simulink model "Rider_Controls_Control"  (R2014b)
settings: configuration reference "Embedded_Configuration" (kept outside this file)
PostLoadFcn:
  | load('Embedded_Config.mat')
model workspace: external: MAT-File C:\Users\Sean\Desktop\Buckeye Current\MagicSimNode\Rider_Controls.mat (data not in the file)
undefined symbols (not defined in the file or in its folder): alpha, BattTemp_Current_x, BattTemp_Current_y, RPM_Max_Current_x, RPM_Max_Current_y, SetPoint
libraries: simulink x1
settings Model: Creator=The MathWorks Inc.  LastModifiedBy=Sean

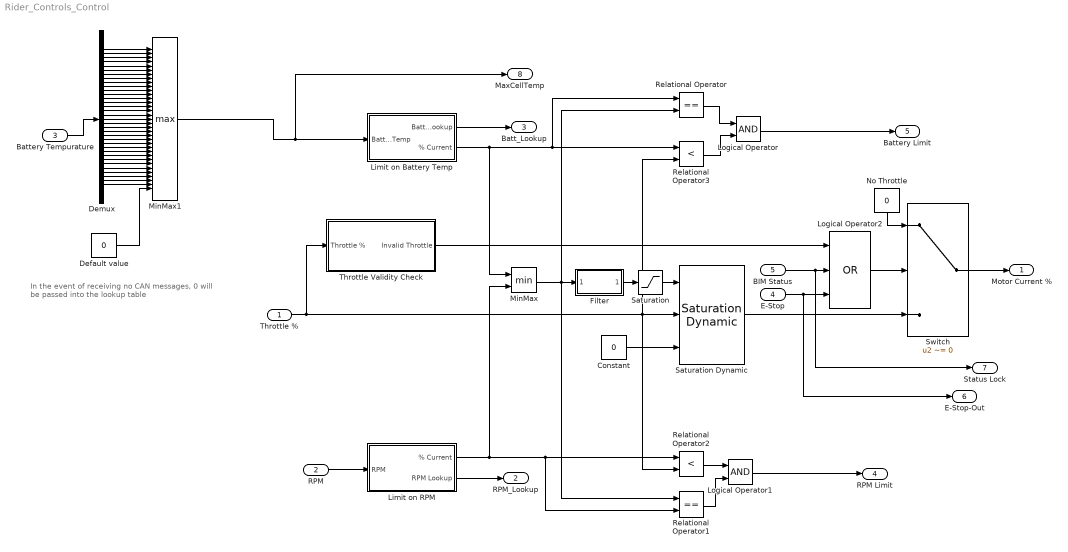
== system Rider_Controls_Control ==
  note: In the event of receiving no CAN messages,
      | 0 will be passed into the lookup table
  Throttle % : Inport  OutDataTypeStr=single  SampleTime=.01
  RPM : Inport  Port=2  OutDataTypeStr=single  SampleTime=.01
  Battery Tempurature : Inport  Port=3  OutDataTypeStr=single  SampleTime=.01
  E-Stop : Inport  Port=4
  BIM Status : Inport  Port=5
  Constant : Constant  Value=0  OutDataTypeStr=single
  Default value : Constant  Value=0  OutDataTypeStr=single
  Demux : Demux  Outputs=34
  Filter : Subsystem
  Limit on Battery Temp : Subsystem
  Limit on RPM : Subsystem
  Logical Operator : Logic  AllPortsSameDT=off  OutDataTypeStr=fixdt(0,16)
  Logical Operator1 : Logic  AllPortsSameDT=off  OutDataTypeStr=fixdt(0,16)
  Logical Operator2 : Logic  Operator=OR  Inputs=3  AllPortsSameDT=off  OutDataTypeStr=fixdt(0,16)
  MinMax : MinMax  Inputs=2
  MinMax1 : MinMax  Function=max  Inputs=35
  No Throttle : Constant  Value=0  OutDataTypeStr=single
  Relational Operator : RelationalOperator  Operator===  OutDataTypeStr=fixdt(0,16)
  Relational Operator1 : RelationalOperator  Operator===  OutDataTypeStr=fixdt(0,16)
  Relational Operator2 : RelationalOperator  Operator=<  OutDataTypeStr=fixdt(0,16)
  Relational Operator3 : RelationalOperator  Operator=<  OutDataTypeStr=fixdt(0,16)
  Saturation : Saturate  UpperLimit=1  LowerLimit=0
  Saturation Dynamic : simulink/Discontinuities/Saturation Dynamic  OutMin=[]  OutMax=[]  OutDataTypeStr=single  OutputDataTypeScalingMode=single  OutDataType=fixdt(1, 16)  OutScaling=2^-10  RndMeth=Nearest  DoSatur=off
  Switch : Switch  Criteria=u2 ~= 0
  Throttle Validity Check : Subsystem
  Motor Current % : Outport
  RPM_Lookup : Outport  Port=2  OutDataTypeStr=single  SampleTime=.01
  Batt_Lookup : Outport  Port=3  OutDataTypeStr=single
  "RPM Limit " : Outport  Port=4
  Battery Limit : Outport  Port=5
  "E-Stop-Out " : Outport  Port=6
  Status Lock : Outport  Port=7
  MaxCellTemp : Outport  Port=8
  wires:
  Throttle %/1 -> Throttle Validity Check/1(Throttle %), Relational Operator2/2, Relational Operator3/2, Saturation Dynamic/2
  Constant/1 -> Saturation Dynamic/3
  Saturation/1 -> Saturation Dynamic/1
  RPM/1 -> Limit on RPM/1(RPM)
  Limit on RPM/2(RPM Lookup) -> RPM_Lookup/1
  Limit on RPM/1(% Current) -> MinMax/2, Relational Operator2/1, Relational Operator1/2
  Limit on Battery Temp/2(% Current) -> MinMax/1, Relational Operator3/1, Relational Operator/1
  MinMax/1 -> Filter/1(Filter In), Relational Operator1/1, Relational Operator/2
  Limit on Battery Temp/1(Batt Temp Lookup) -> Batt_Lookup/1
  Relational Operator3/1 -> Logical Operator/2
  Relational Operator/1 -> Logical Operator/1
  Relational Operator2/1 -> Logical Operator1/1
  Relational Operator1/1 -> Logical Operator1/2
  No Throttle/1 -> Switch/1
  Saturation Dynamic/1 -> Switch/3
  Throttle Validity Check/1(Invalid Throttle) -> Logical Operator2/1
  Switch/1 -> Motor Current %/1
  BIM Status/1 -> Logical Operator2/2, Status Lock/1
  Battery Tempurature/1 -> Demux/1
  Demux/1 -> MinMax1/1
  Demux/2 -> MinMax1/2
  Demux/3 -> MinMax1/3
  Demux/4 -> MinMax1/4
  Demux/5 -> MinMax1/5
  Demux/6 -> MinMax1/6
  Demux/7 -> MinMax1/7
  Demux/8 -> MinMax1/8
  Demux/9 -> MinMax1/9
  Demux/10 -> MinMax1/10
  Demux/11 -> MinMax1/11
  Demux/12 -> MinMax1/12
  Demux/13 -> MinMax1/13
  Demux/14 -> MinMax1/14
  Demux/15 -> MinMax1/15
  Demux/16 -> MinMax1/16
  Demux/17 -> MinMax1/17
  Demux/18 -> MinMax1/18
  Demux/19 -> MinMax1/19
  Demux/20 -> MinMax1/20
  Demux/21 -> MinMax1/21
  Demux/22 -> MinMax1/22
  Demux/23 -> MinMax1/23
  Demux/24 -> MinMax1/24
  Demux/25 -> MinMax1/25
  Demux/26 -> MinMax1/26
  Demux/27 -> MinMax1/27
  Demux/28 -> MinMax1/28
  Demux/29 -> MinMax1/29
  Demux/30 -> MinMax1/30
  Demux/31 -> MinMax1/31
  Demux/32 -> MinMax1/32
  Demux/33 -> MinMax1/33
  Demux/34 -> MinMax1/34
  MinMax1/1 -> MaxCellTemp/1, Limit on Battery Temp/1(Battery Temp)
  E-Stop/1 -> "E-Stop-Out "/1, Logical Operator2/3
  Logical Operator2/1 -> Switch/2
  Logical Operator/1 -> Battery Limit/1
  Logical Operator1/1 -> "RPM Limit "/1
  Default value/1 -> MinMax1/35
  Filter/1(Filter Out) -> Saturation/1

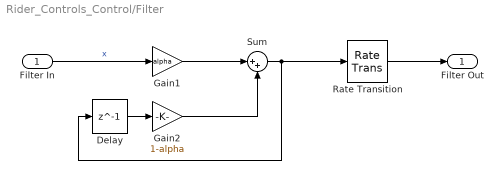
== system Rider_Controls_Control/Filter ==
  Filter In : Inport
  Delay : Delay  DelayLength=1
  Gain1 : Gain  Gain=alpha
  Gain2 : Gain  Gain=1-alpha
  Rate Transition : RateTransition  OutPortSampleTime=.01
  Sum : Sum  Inputs=|++  OutDataTypeStr=single
  Filter Out : Outport  SampleTime=.01
  wires:
  Rate Transition/1 -> Filter Out/1
  Sum/1 -> Delay/1, Rate Transition/1
  Gain2/1 -> Sum/2
  Delay/1 -> Gain2/1
  Gain1/1 -> Sum/1
  Filter In/1 -> Gain1/1  "x"

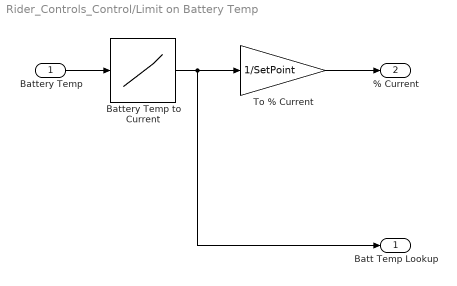
== system Rider_Controls_Control/Limit on Battery Temp ==
  Battery Temp : Inport
  Battery Temp to Current : Lookup_n-D  NumberOfTableDimensions=1  BreakpointsForDimension1=BattTemp_Current_x  BreakpointsForDimension1DataTypeStr=single  IndexSearchMethod=Linear search  BeginIndexSearchUsingPreviousIndexResult=on  Table=BattTemp_Current_y  TableDataTypeStr=single  IntermediateResultsDataTypeStr=single  RemoveProtectionInput=on  InternalRulePriority=Speed  OutDataTypeStr=single  RndMeth=Simplest  FractionDataTypeStr=single  InputSameDT=on
  To % Current : Gain  Gain=1/SetPoint  OutDataTypeStr=single  RndMeth=Nearest
  Batt Temp Lookup : Outport
  % Current : Outport  Port=2
  wires:
  To % Current/1 -> % Current/1
  Battery Temp/1 -> Battery Temp to Current/1
  Battery Temp to Current/1 -> To % Current/1, Batt Temp Lookup/1

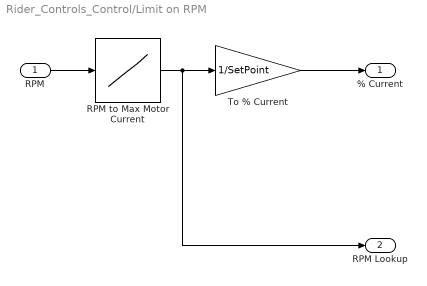
== system Rider_Controls_Control/Limit on RPM ==
  RPM : Inport
  RPM to Max Motor Current : Lookup_n-D  NumberOfTableDimensions=1  BreakpointsForDimension1=RPM_Max_Current_x  BreakpointsForDimension1DataTypeStr=single  IndexSearchMethod=Linear search  BeginIndexSearchUsingPreviousIndexResult=on  Table=RPM_Max_Current_y  TableDataTypeStr=single  IntermediateResultsDataTypeStr=single  RemoveProtectionInput=on  InternalRulePriority=Speed  OutDataTypeStr=single  RndMeth=Simplest  FractionDataTypeStr=single  InputSameDT=on
  To % Current : Gain  Gain=1/SetPoint  OutDataTypeStr=single  RndMeth=Nearest
  % Current : Outport
  RPM Lookup : Outport  Port=2
  wires:
  RPM to Max Motor Current/1 -> RPM Lookup/1, To % Current/1
  RPM/1 -> RPM to Max Motor Current/1
  To % Current/1 -> % Current/1

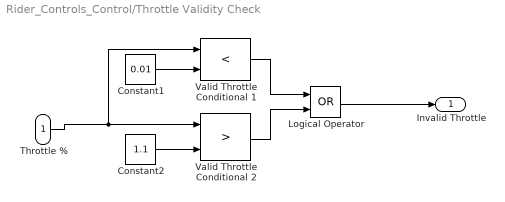
== system Rider_Controls_Control/Throttle Validity Check ==
  Throttle % : Inport
  Constant1 : Constant  Value=0.01
  Constant2 : Constant  Value=1.1
  Logical Operator : Logic  Operator=OR  AllPortsSameDT=off  OutDataTypeStr=fixdt(0,16)
  Valid Throttle Conditional 1 : RelationalOperator  Operator=<  OutDataTypeStr=boolean
  Valid Throttle Conditional 2 : RelationalOperator  Operator=>  OutDataTypeStr=boolean
  Invalid Throttle : Outport
  wires:
  Throttle %/1 -> Valid Throttle Conditional 1/1, Valid Throttle Conditional 2/1
  Constant1/1 -> Valid Throttle Conditional 1/2
  Constant2/1 -> Valid Throttle Conditional 2/2
  Valid Throttle Conditional 1/1 -> Logical Operator/1
  Valid Throttle Conditional 2/1 -> Logical Operator/2
  Logical Operator/1 -> Invalid Throttle/1
